simulink model "H175_Stage_01_Anode_Cathode"  (R2023a)
settings: Solver=VariableStepAuto  StartTime=0.0  StopTime=500  RelTol=1e-3
values from neighbouring files (symbols this model uses):
  anode_tube_D = 0.01    [All_Properties.mat]    (also in anode_subsystem_parameters.m; environment_parameters.m)
  D = 0.01    [All_Properties.mat]    (also in anode_subsystem_parameters.m)
  densityHydrogen = 0.0899    [All_Properties.mat]    (also in Valve_Init.m; anode_subsystem_parameters.m)
  Fischer_EMTC120K_supplier_mdot_TLU = [33.385172 57.11265182 82.35238332 173.9183787 230.2050798 50.1655574 86.1774137 122.96585 210.0188714 258.8737112 70.20710678 115.3896052 ... (25 elements, 5x5)]    [All_Properties.mat]    (also in cathode_subsystem_parameters.m = [33.385172 50.1655574 70.20710678 87.4902972 105.3161257)
  Fischer_EMTC120K_supplier_pr_TLU = [2.452176848 3.067593046 4.01020547 5.11549365 6.10066015 2.450765612 3.07166407 4.0616557 5.112468546 6.108742034 2.432340262 3.033516574 ... (25 elements, 5x5)]    [All_Properties.mat]    (also in cathode_subsystem_parameters.m = [2.452176848 2.450765612 2.432340262 2.407245766 2.37067916)
  Kv_VL6112 = 0.8    [All_Properties.mat]    (also in anode_subsystem_parameters.m)
  N2_T = [-56.55 -50 -40 -30 -20 -10 -5 -4 -3 -2 -1 0 ... (52 elements, 1x52)]    [All_Properties.mat]    (also in anode_subsystem_parameters.m = [-56.55 -50 -40 -30 -20 -10 -5 -4 -3 -2 -1 0 1 2 3 4 5 10 20; environment_parameters.m = [-56.55, -50:10:-10, -5:1:5, 10:10:350]; stack_model_harness_parameters.m = [-56.55, -50:10:-10, -5:1:5, 10:10:350])
  p_range = 0.005    [All_Properties.mat]    (also in anode_subsystem_parameters.m)
  r_max = 0.2    [All_Properties.mat]    (also in anode_subsystem_parameters.m)
  r_min = 0.0001    [All_Properties.mat]    (also in anode_subsystem_parameters.m)
  responseTimeValve = 0.013    [All_Properties.mat]    (also in anode_subsystem_parameters.m)
undefined symbols (not defined in the file or in its folder): sigbuilder_block
libraries: fl_lib x168, nesl_utility x116, SimscapeFluids_lib x8, slpidlib x5, simulink x1
(part 2 of 8)

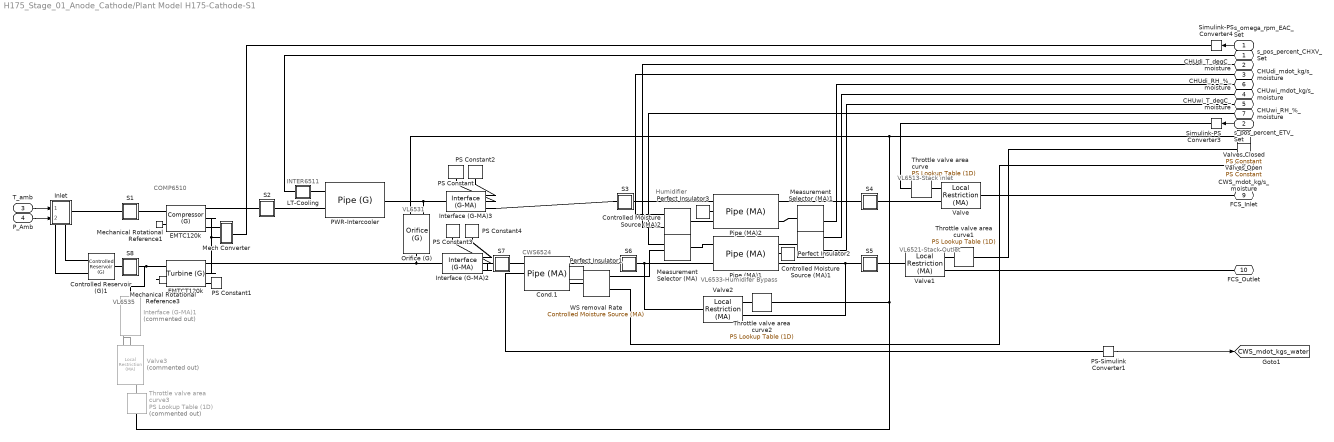
== system H175_Stage_01_Anode_Cathode/Plant Model H175-Cathode-S1 ==
  note: Humidifier
  note: COMP6510
  note: INTER6511
  note: VL6531
  note: VL6513-Stack inlet
  note: VL6521-Stack Outlet
  note: VL6533-Humidifer Bypass
  note: VL6535
  note: CWS6524
  s_omega_rpm_EAC_Set : Inport
  s_pos_percent_ETV_Set : Inport  Port=2
  T_amb : Inport  Port=3
  P_Amb : Inport  Port=4
  Cond.1 : fl_lib/Moist Air/Elements/Pipe (MA)  length=1 m  area=1 m^2  Dh=.1 m  length_add=.1 m  roughness=15e-6 m  Re_lam=2000  Re_tur=4000  shape_factor=64  Nu_lam=3.66  wall_condensation=simscape.enum.onoff.on  RH_ws=.2  time_constant=1e-3 s  moisture_trace_gas_source=foundation.enum.moisture_trace_gas_source.controlled  moisture_source_spec=foundation.enum.moisture_source_spec.vapor  moisture_mass_flow=0 kg/s  moisture_temperature_spec=foundation.enum.temperature_spec.atmospheric  moisture_temperature=293.15 K  trace_gas_mass_flow=0 kg/s  trace_gas_temperature_spec=foundation.enum.temperature_spec.atmospheric  trace_gas_temperature=293.15 K  p_I_specify=off  p_I_priority=High  p_I=0.101325 MPa  p_I_nominal_specify=off  p_I_nominal_unit=MPa  p_I_nominal_value=1  T_I_specify=off  T_I_priority=High  T_I=293.15 K  T_I_nominal_specify=off  T_I_nominal_unit=K  T_I_nominal_value=1  RH_I_specify=off  RH_I_priority=High  RH_I=0  RH_I_nominal_specify=off  RH_I_nominal_unit=1  RH_I_nominal_value=1  x_w_I_specify=off  x_w_I_priority=None  x_w_I=0  x_w_I_nominal_specify=off  x_w_I_nominal_unit=1  x_w_I_nominal_value=1  y_w_I_specify=off  y_w_I_priority=None  y_w_I=0  y_w_I_nominal_specify=off  y_w_I_nominal_unit=1  y_w_I_nominal_value=1  HR_I_specify=off  HR_I_priority=None  HR_I=0  HR_I_nominal_specify=off  HR_I_nominal_unit=1  HR_I_nominal_value=1  x_g_I_specify=off  x_g_I_priority=High  x_g_I=0  x_g_I_nominal_specify=off  x_g_I_nominal_unit=1  x_g_I_nominal_value=1  y_g_I_specify=off  y_g_I_priority=None  y_g_I=0  y_g_I_nominal_specify=off  y_g_I_nominal_unit=1  y_g_I_nominal_value=1
      settings: InternalSimscapePortConfiguration="{\"Bottom\":[],\"Left\":[{\"id\":\"A\",\"label\":\"A\",\"type\":\"foundation.moist_air.moist_air\"},{\"id\":\"H\",\"label\":\"H\",\"type\":\"foundation.thermal.thermal\"},{\"id\":\"S\",\"label\":\"S\",\"type\":\"foundation.moist_air.moist_air_source\"}],\"Right\":[{\"id\":\"B\",\"label\":\"B\",\"type\":\"foundation.moist_air.moist_air\"},{\"id\":\"W\",\"label\":\"W\",\"type\":\"output\"},{\"id\":\"F\",\"label\":\"F\",\"type\":\"output\"}],\"Top\":[]}"
  Controlled Moisture Source (MA)1 : fl_lib/Moist Air/Sources/Moisture & Trace Gas Sources/Controlled Moisture Source (MA)  moisture_source_spec=foundation.enum.moisture_source_spec.vapor  Phi_S_specify=off  Phi_S_priority=None  Phi_S=0 kW  Phi_S_nominal_specify=off  Phi_S_nominal_unit=kW  Phi_S_nominal_value=1  mdot_w_S_specify=off  mdot_w_S_priority=None  mdot_w_S=0 kg/s  mdot_w_S_nominal_specify=off  mdot_w_S_nominal_unit=kg/s  mdot_w_S_nominal_value=1
      settings: InternalSimscapePortConfiguration="{\"Bottom\":[],\"Left\":[{\"id\":\"S\",\"label\":\"S\",\"type\":\"foundation.moist_air.moist_air_source\"}],\"Right\":[{\"id\":\"M\",\"label\":\"M\",\"type\":\"input\"},{\"id\":\"T\",\"label\":\"T\",\"type\":\"input\"}],\"Top\":[]}"
  Controlled Moisture Source (MA)2 : fl_lib/Moist Air/Sources/Moisture & Trace Gas Sources/Controlled Moisture Source (MA)  moisture_source_spec=foundation.enum.moisture_source_spec.vapor  Phi_S_specify=off  Phi_S_priority=None  Phi_S=0 kW  Phi_S_nominal_specify=off  Phi_S_nominal_unit=kW  Phi_S_nominal_value=1  mdot_w_S_specify=off  mdot_w_S_priority=None  mdot_w_S=0 kg/s  mdot_w_S_nominal_specify=off  mdot_w_S_nominal_unit=kg/s  mdot_w_S_nominal_value=1
      settings: InternalSimscapePortConfiguration="{\"Bottom\":[],\"Left\":[{\"id\":\"S\",\"label\":\"S\",\"type\":\"foundation.moist_air.moist_air_source\"}],\"Right\":[{\"id\":\"M\",\"label\":\"M\",\"type\":\"input\"},{\"id\":\"T\",\"label\":\"T\",\"type\":\"input\"}],\"Top\":[]}"
  Controlled Reservoir (G)1 : fl_lib/Gas/Elements/Controlled Reservoir (G)  area_A=0.002 m^2
      settings: InternalSimscapePortConfiguration="{\"Bottom\":[],\"Left\":[{\"id\":\"A\",\"label\":\"A\",\"type\":\"foundation.gas.gas\"}],\"Right\":[{\"id\":\"T_in\",\"label\":\"T\",\"type\":\"input\"},{\"id\":\"p_in\",\"label\":\"P\",\"type\":\"input\"}],\"Top\":[]}"
  EMTC120k : SimscapeFluids_lib/Gas/Turbomachinery/Compressor (G)  parameterization=fluids.gas.turbomachinery.enum.CompressorParameterization.Tabulated  NDes=10000 rpm  piDes=7.5  mdotDes=33 kg/s  efficiencyType=fluids.gas.turbomachinery.enum.EfficiencyType.Analytical  efficiencyValue=0.8  etaMax=0.887  etaMin=0.5  mdotMaxEff=30 kg/s  piMaxEff=7  omega_TLU=Fischer_EMTC120K_supplier_omega_TLU rpm  beta_TLU=Fischer_EMTC120K_supplier_beta_TLU  pr_TLU=Fischer_EMTC120K_supplier_pr_TLU/2  mdot_TLU=Fischer_EMTC120K_supplier_mdot_TLU/2 g/s  eta_TLU=Fischer_EMTC120K_supplier_eta_TLU  SMFault=simscape.enum.assert.action.none  a=1.5  b=5  k=0.03  c=3  d=4  cCap=15  dCap=1.0  p_reference=0.101325 MPa  T_reference=288.15 K  mechanical_efficiency=0.98  area_A=.002 m^2  area_B=.002 m^2
      settings: LogSimulationData=on  InternalSimscapePortConfiguration="{\"Bottom\":[],\"Left\":[{\"id\":\"A\",\"label\":\"A\",\"type\":\"foundation.gas.gas\"},{\"id\":\"C\",\"label\":\"C\",\"type\":\"foundation.mechanical.rotational.rotational\"}],\"Right\":[{\"id\":\"B\",\"label\":\"B\",\"type\":\"foundation.gas.gas\"},{\"id\":\"R\",\"label\":\"R\",\"type\":\"foundation.mechanical.rotational.rotational\"},{\"id\":\"SM\",\"label\":\"SM\",\"type\":\"output\"}],\"Top\":[]}"
  EMTCT120k : SimscapeFluids_lib/Gas/Turbomachinery/Turbine (G)  parameterization=fluids.gas.turbomachinery.enum.TurbineParameterization.Tabulated1D  omega_TLU_2=[31000, 45000, 60000, 75000, 90000, 105000, 120000] rpm  variable_nozzle=true  min_nozzle_opening=1e-3  max_nozzle_opening=1  pr_nom=2  mdot_nom=0.08 kg/s  pr_mdot_TLU=[1.1667,1.405,1.791,2.18,2.5194]  mdot_TLU=[.0527,.08728,.1276,.1668,.1927] kg/s  pr_mdot_TLU_2=[1.217, 1.285, 1.323, 1.363, 1.402, 1.427, 1.495, 1.545, 1.6, 1.687, 1.747, 1.8074; 1.231, 1.302, 1.356, 1.404, 1.443, 1.473, 1.525, 1.577, 1.635, 1.709, 1.782, 1.845; 1.242, 1.328, 1.388, 1.437, 1.528, 1.617, 1.704, 1.811, 1.915, 1.979, 2.053, 2.1226; 1.244, 1.339, 1.417, 1.465, 1.528, 1.584, 1.692, 1.787, 1.899, 2, 2.075, 2.1492; 1.245, 1.34, 1.425, 1.492, 1.546, 1.684, 1.748, 1.882, 1.987, 2.084, 2.167, 2.2458; 1.251, 1.345, 1.442, 1.521, 1.596, 1.692, 1.849, 1.972, 2.1, 2.173, 2.259, 2.3424; 1.248, 1.348, 1.447, 1.516, 1.581, 1.651, 1.749, 1.839, 1.93, 2.024, 2.154, 2.242]  mdot_TLU_2=[40.403, 44.417, 46.653, 47.966, 48.97, 49.544, 50.001, 50.081, 50.086, 50.095, 50.09, 50.0922; 40.044, 43.754, 46.125, 47.626, 48.513, 49.105, 49.481, 49.58, 49.597, 49.624, 49.638, 49.633; 39.941, 43.795, 46.017, 47.335, 48.795, 49.199, 49.279, 49.27, 49.248, 49.23, 49.255, 49.2428; 39.896, 43.512, 45.914, 47.061, 48.011, 48.558, 48.943, 49.042, 49.069, 49.01, 49.046, 49.0266; 39.524, 42.934, 45.686, 46.743, 47.715, 48.67, 48.777, 48.836, 48.876, 48.836, 48.845, 48.8184; 39.439, 43.01, 45.556, 46.801, 47.792, 48.388, 48.634, 48.67, 48.639, 48.647, 48.625, 48.5912; 39.502, 42.849, 45.336, 46.385, 47.312, 47.877, 48.222, 48.397, 48.459, 48.482, 48.455, 48.414] kg/s  efficiency_constant=.954  pr_eta_TLU=[1.1667,1.405,1.791,2.18,2.5194]  eta_TLU=[0.6804,.76609,.7634,.7426,.72]  pr_eta_TLU_2=[1.224, 1.246, 1.292, 1.387, 1.457, 1.534, 1.61, 1.686, 1.743, 1.79, 1.871, 1.914; 1.237, 1.25, 1.28, 1.369, 1.459, 1.553, 1.629, 1.716, 1.799, 1.846, 1.927, 1.97; 1.241, 1.255, 1.283, 1.326, 1.401, 1.509, 1.591, 1.704, 1.806, 1.913, 1.994, 2.037; 1.25, 1.265, 1.308, 1.364, 1.456, 1.532, 1.637, 1.739, 1.851, 1.934, 2.042, 2.085; 1.281, 1.314, 1.371, 1.425, 1.498, 1.574, 1.647, 1.749, 1.878, 1.979, 2.091, 2.18; 1.252, 1.328, 1.425, 1.544, 1.642, 1.757, 1.873, 2.005, 2.1, 2.204, 2.248, 2.28; 1.382, 1.43, 1.495, 1.586, 1.688, 1.791, 1.887, 1.99, 2.079, 2.158, 2.249, 2.36]  eta_TLU_2=[.72, .754, .759, .739, .714, .679, .643, .603, .554, .524, .494, .48; .716, .757, .794, .819, .812, .788, .761, .728, .692, .662, .632, .618; .629, .691, .775, .831, .858, .869, .859, .842, .816, .782, .752, .738; .594, .668, .757, .804, .857, .883, .892, .893, .884, .865, .835, .821; .664, .72, .779, .823, .858, .883, .897, .905, .904, .896, .883, .868; .559, .61, .673, .741, .788, .835, .869, .895, .908, .899, .854, .751; .718, .785, .824, .855, .882, .9, .908, .906, .884, .857, .804, .701]  p_reference=1.8 bar  T_reference=85 degC  mechanical_efficiency=0.98  area_A=0.002 m^2  area_B=0.002 m^2
      settings: LogSimulationData=on  InternalSimscapePortConfiguration="{\"Bottom\":[],\"Left\":[{\"id\":\"A\",\"label\":\"A\",\"type\":\"foundation.gas.gas\"},{\"id\":\"R\",\"label\":\"R\",\"type\":\"foundation.mechanical.rotational.rotational\"},{\"id\":\"VN\",\"label\":\"VN\",\"type\":\"input\"}],\"Right\":[{\"id\":\"B\",\"label\":\"B\",\"type\":\"foundation.gas.gas\"},{\"id\":\"C\",\"label\":\"C\",\"type\":\"foundation.mechanical.rotational.rotational\"}],\"Top\":[]}"
  Inlet : Subsystem
      settings: PortSchema="{\"entries\":[{\"content\":{\"sides\":[{\"content\":{\"connectorIds\":[\"In1\",\"In2\"]},\"type\":\"ConnectorPlacement.EquallySpacedRectSide\",\"uuid\":\"383c8b90-d22b-483c-be09-d78d9bde0881\"},{\"content\":{\"connectorIds\":[\"RConn1\"],\"side\":\"RIGHT\"},\"type\":\"ConnectorPlacement.EquallySpacedRectSide\",\"uuid\":\"3dc3e004-4331-4c40-8051-329aa9250422\"},{\"content\":{\"side\":\"TOP\"},\"type\":\"ConnectorPlacement.EquallySpacedRectSide\",\"uuid\":\"aff35d8f-ac03-451a-b72e-dc7bd89924e8\"},{\"content\":{\"connectorIds\":[\"RConn2\",\"RConn3\"],\"side\":\"BOTTOM\"},\"type\":\"ConnectorPlacement.EquallySpacedRectSide\",\"uuid\":\"82493911-a5c4-468a-a003-983b92ffd105\"}]},\"type\":\"ConnectorPlacement.EquallySpacedConnector\",\"uuid\":\"d9a1e9aa-22f5-4e42-bf15-8a8ecd9f58f9\"}],\"packageUris\":[\"http://schema.mathworks.com/mf0/Connector/R2020b\"],\"version\":\"1.0\"}"
  Interface (G-MA)1 : SimscapeFluids_lib/Fluid Network Interfaces/Interface (G-MA)  Commented=on  interface_type=foundation.enum.constant_controlled.controlled  moisture_spec=foundation.enum.moisture_spec.relative_humidity  RH_interface=0.5  x_w_interface=0.01  y_w_interface=0.01  HR_interface=0.01  Tw_interface=287 K  trace_gas_spec=foundation.enum.trace_gas_spec.mass_fraction  x_g_interface=1  y_g_interface=0.001  RH_ws=1  area=0.01 m^2  input_error_spec=foundation.enum.input_range_error.warn
      settings: InternalSimscapePortConfiguration="{\"Bottom\":[{\"id\":\"W\",\"label\":\"W\",\"type\":\"input\"},{\"id\":\"TG\",\"label\":\"TG\",\"type\":\"input\"}],\"Left\":[{\"id\":\"G\",\"label\":\"G\",\"type\":\"foundation.gas.gas\"}],\"Right\":[{\"id\":\"MA\",\"label\":\"MA\",\"type\":\"foundation.moist_air.moist_air\"}],\"Top\":[]}"
  Interface (G-MA)2 : SimscapeFluids_lib/Fluid Network Interfaces/Interface (G-MA)  interface_type=foundation.enum.constant_controlled.controlled  moisture_spec=foundation.enum.moisture_spec.relative_humidity  RH_interface=0.5  x_w_interface=0.01  y_w_interface=0.01  HR_interface=0.01  Tw_interface=287 K  trace_gas_spec=foundation.enum.trace_gas_spec.mass_fraction  x_g_interface=1  y_g_interface=0.001  RH_ws=1  area=0.01 m^2  input_error_spec=foundation.enum.input_range_error.warn
      settings: InternalSimscapePortConfiguration="{\"Bottom\":[{\"id\":\"W\",\"label\":\"W\",\"type\":\"input\"},{\"id\":\"TG\",\"label\":\"TG\",\"type\":\"input\"}],\"Left\":[{\"id\":\"G\",\"label\":\"G\",\"type\":\"foundation.gas.gas\"}],\"Right\":[{\"id\":\"MA\",\"label\":\"MA\",\"type\":\"foundation.moist_air.moist_air\"}],\"Top\":[]}"
  Interface (G-MA)3 : SimscapeFluids_lib/Fluid Network Interfaces/Interface (G-MA)  interface_type=foundation.enum.constant_controlled.controlled  moisture_spec=foundation.enum.moisture_spec.relative_humidity  RH_interface=0.5  x_w_interface=0.01  y_w_interface=0.01  HR_interface=0.01  Tw_interface=287 K  trace_gas_spec=foundation.enum.trace_gas_spec.mass_fraction  x_g_interface=1  y_g_interface=0.001  RH_ws=1  area=0.002 m^2  input_error_spec=foundation.enum.input_range_error.warn
      settings: InternalSimscapePortConfiguration="{\"Bottom\":[{\"id\":\"W\",\"label\":\"W\",\"type\":\"input\"},{\"id\":\"TG\",\"label\":\"TG\",\"type\":\"input\"}],\"Left\":[{\"id\":\"G\",\"label\":\"G\",\"type\":\"foundation.gas.gas\"}],\"Right\":[{\"id\":\"MA\",\"label\":\"MA\",\"type\":\"foundation.moist_air.moist_air\"}],\"Top\":[]}"
  LT-Cooling : Subsystem
  Measurement Selector (MA) : fl_lib/Moist Air/Sensors/Measurement Selector (MA)  moisture_spec=foundation.enum.moisture_spec.relative_humidity  trace_gas_spec=foundation.enum.trace_gas_spec.mole_fraction
  Measurement Selector (MA)1 : fl_lib/Moist Air/Sensors/Measurement Selector (MA)  moisture_spec=foundation.enum.moisture_spec.relative_humidity  trace_gas_spec=foundation.enum.trace_gas_spec.mole_fraction
  Mech Converter : Subsystem
  Mechanical Rotational Reference1 : fl_lib/Mechanical/Rotational Elements/Mechanical Rotational Reference
  Mechanical Rotational Reference3 : fl_lib/Mechanical/Rotational Elements/Mechanical Rotational Reference
  Orifice (G) : SimscapeFluids_lib/Gas/Valves & Orifices/Orifice (G)  orifice_type=foundation.enum.constant_variable.variable  orifice_parameterization=fluids.gas.valves_orifices.enum.OrificeParameterization.Area  opening_characteristic=fluids.gas.valves_orifices.enum.OpeningCharacteristics.Tabulated  Cv_constant=4  Cv_max=.369  L_Cv_TLU=0 : 0.2 : 1  Cv_TLU=[1e-06, .8, 1.6, 2.4, 3.2, 4]  xT_Cv=0.35  Kv_constant=3.6  Kv_max=50  L_Kv_TLU=[0,.15, .25, .35, .5, 1]  Kv_TLU=[1,27.76,115.14,223.57,336.62,462.54]  xT_Kv=.027  C_constant=12 l/(bar*s)  B_crit_constant=0.3  C_max=40 l/(bar*s)  B_crit_linear=0.25  L_C_TLU=0 : 0.2 : 1  C_TLU=[1e-05, 2.4, 4.8, 7.2, 9.6, 12] l/(bar*s)  B_crit_TLU=0.3 * ones(1, 6)  m=0.5  T_ref_C=293.15 K  rho_ref_C=1.185 kg/m^3  orifice_area_constant=1e-4 m^2  orifice_area_max=0.00152 m^2  L_orifice_area_TLU=[0.111111111,0.222222222,0.333333333,0.444444444,0.555555556,0.666666667,0.777777778,0.888888889,1]  orifice_area_TLU=[2.00E-08,9.00E-08,0.0002,0.00035,0.00055,0.00077,0.00101,0.00125,0.00153] m^2  Cd=.64  leakage_fraction=0.03185  smoothing_factor=0.01  B_lam=9.44E-01  area=0.002 m^2
      settings: InternalSimscapePortConfiguration="{\"Bottom\":[],\"Left\":[{\"id\":\"A\",\"label\":\"A\",\"type\":\"foundation.gas.gas\"},{\"id\":\"L\",\"label\":\"L\",\"type\":\"input\"}],\"Right\":[{\"id\":\"B\",\"label\":\"B\",\"type\":\"foundation.gas.gas\"}],\"Top\":[]}"
  PS Constant : fl_lib/Physical Signals/Sources/PS Constant  constant=.2
  PS Constant1 : fl_lib/Physical Signals/Sources/PS Constant  constant=1
  PS Constant2 : fl_lib/Physical Signals/Sources/PS Constant  constant=.001
  PS Constant3 : fl_lib/Physical Signals/Sources/PS Constant  constant=.3
  PS Constant4 : fl_lib/Physical Signals/Sources/PS Constant  constant=.001
  PS-Simulink Converter1 : nesl_utility/PS-Simulink Converter  PhysicalDomain=network_engine_domain  SubClassName=ps_output  LeftPortType=input  RightPortType=output  PseudoPeriodic=off  Frequencies=[]  VectorFormat=inherit  Unit=inherit  AffineConversion=off
  PWR-Intercooler : fl_lib/Gas/Elements/Pipe (G)  length=1 m  area=1 m^2  Dh=0.1 m  length_add=.2 m  roughness=15e-14 m  Re_lam=2000  Re_tur=4000  shape_factor=3.66  Nu_lam=150  p_I_specify=off  p_I_priority=High  p_I=1.8 bar  p_I_nominal_specify=off  p_I_nominal_unit=MPa  p_I_nominal_value=.1  T_I_specify=off  T_I_priority=High  T_I=293.15 K  T_I_nominal_specify=off  T_I_nominal_unit=K  T_I_nominal_value=1  rho_I_specify=off  rho_I_priority=None  rho_I=1.2 kg/m^3  rho_I_nominal_specify=off  rho_I_nominal_unit=kg/m^3  rho_I_nominal_value=1
      settings: LogSimulationData=on
  Perfect Insulator1 : fl_lib/Thermal/Thermal Elements/Perfect Insulator  T_specify=off  T_priority=None  T=293.15 K  T_nominal_specify=off  T_nominal_unit=K  T_nominal_value=1
  Perfect Insulator2 : fl_lib/Thermal/Thermal Elements/Perfect Insulator  T_specify=off  T_priority=None  T=0 K  T_nominal_specify=off  T_nominal_unit=K  T_nominal_value=1
  Perfect Insulator3 : fl_lib/Thermal/Thermal Elements/Perfect Insulator  T_specify=off  T_priority=None  T=0 K  T_nominal_specify=off  T_nominal_unit=K  T_nominal_value=1
  Pipe (MA)1 : fl_lib/Moist Air/Elements/Pipe (MA)  length=0.25 m  area=pi*0.05^2/4 m^2  Dh=0.05 m  length_add=0.1 m  roughness=15e-6 m  Re_lam=2000  Re_tur=4000  shape_factor=64  Nu_lam=3.66  wall_condensation=simscape.enum.onoff.off  RH_ws=1  time_constant=1e-3 s  moisture_trace_gas_source=foundation.enum.moisture_trace_gas_source.controlled  moisture_source_spec=foundation.enum.moisture_source_spec.vapor  moisture_mass_flow=0 kg/s  moisture_temperature_spec=foundation.enum.temperature_spec.atmospheric  moisture_temperature=293.15 K  trace_gas_mass_flow=0 kg/s  trace_gas_temperature_spec=foundation.enum.temperature_spec.atmospheric  trace_gas_temperature=293.15 K  p_I_specify=off  p_I_priority=High  p_I=env_p MPa  p_I_nominal_specify=off  p_I_nominal_unit=MPa  p_I_nominal_value=1  T_I_specify=off  T_I_priority=High  T_I=env_T degC  T_I_nominal_specify=off  T_I_nominal_unit=K  T_I_nominal_value=1  RH_I_specify=off  RH_I_priority=High  RH_I=env_RH  RH_I_nominal_specify=off  RH_I_nominal_unit=1  RH_I_nominal_value=1  x_w_I_specify=off  x_w_I_priority=None  x_w_I=0  x_w_I_nominal_specify=off  x_w_I_nominal_unit=1  x_w_I_nominal_value=1  y_w_I_specify=off  y_w_I_priority=None  y_w_I=0  y_w_I_nominal_specify=off  y_w_I_nominal_unit=1  y_w_I_nominal_value=1  HR_I_specify=off  HR_I_priority=None  HR_I=0  HR_I_nominal_specify=off  HR_I_nominal_unit=1  HR_I_nominal_value=1  x_g_I_specify=off  x_g_I_priority=None  x_g_I=0  x_g_I_nominal_specify=off  x_g_I_nominal_unit=1  x_g_I_nominal_value=1  y_g_I_specify=off  y_g_I_priority=High  y_g_I=env_yO2  y_g_I_nominal_specify=off  y_g_I_nominal_unit=1  y_g_I_nominal_value=1
      settings: InternalSimscapePortConfiguration="{\"Bottom\":[],\"Left\":[{\"id\":\"A\",\"label\":\"A\",\"type\":\"foundation.moist_air.moist_air\"},{\"id\":\"H\",\"label\":\"H\",\"type\":\"foundation.thermal.thermal\"},{\"id\":\"S\",\"label\":\"S\",\"type\":\"foundation.moist_air.moist_air_source\"}],\"Right\":[{\"id\":\"B\",\"label\":\"B\",\"type\":\"foundation.moist_air.moist_air\"},{\"id\":\"W\",\"label\":\"W\",\"type\":\"output\"},{\"id\":\"F\",\"label\":\"F\",\"type\":\"output\"}],\"Top\":[]}"
  Pipe (MA)2 : fl_lib/Moist Air/Elements/Pipe (MA)  length=0.25 m  area=pi*0.05^2/4 m^2  Dh=0.05 m  length_add=0.1 m  roughness=15e-6 m  Re_lam=2000  Re_tur=4000  shape_factor=64  Nu_lam=3.66  wall_condensation=simscape.enum.onoff.off  RH_ws=1  time_constant=1e-3 s  moisture_trace_gas_source=foundation.enum.moisture_trace_gas_source.controlled  moisture_source_spec=foundation.enum.moisture_source_spec.vapor  moisture_mass_flow=0 kg/s  moisture_temperature_spec=foundation.enum.temperature_spec.atmospheric  moisture_temperature=293.15 K  trace_gas_mass_flow=0 kg/s  trace_gas_temperature_spec=foundation.enum.temperature_spec.atmospheric  trace_gas_temperature=293.15 K  p_I_specify=off  p_I_priority=High  p_I=env_p MPa  p_I_nominal_specify=off  p_I_nominal_unit=MPa  p_I_nominal_value=1  T_I_specify=on  T_I_priority=High  T_I=env_T degC  T_I_nominal_specify=off  T_I_nominal_unit=K  T_I_nominal_value=1  RH_I_specify=on  RH_I_priority=High  RH_I=env_RH  RH_I_nominal_specify=off  RH_I_nominal_unit=1  RH_I_nominal_value=1  x_w_I_specify=off  x_w_I_priority=None  x_w_I=0  x_w_I_nominal_specify=off  x_w_I_nominal_unit=1  x_w_I_nominal_value=1  y_w_I_specify=off  y_w_I_priority=None  y_w_I=0  y_w_I_nominal_specify=off  y_w_I_nominal_unit=1  y_w_I_nominal_value=1  HR_I_specify=off  HR_I_priority=None  HR_I=0  HR_I_nominal_specify=off  HR_I_nominal_unit=1  HR_I_nominal_value=1  x_g_I_specify=off  x_g_I_priority=None  x_g_I=0  x_g_I_nominal_specify=off  x_g_I_nominal_unit=1  x_g_I_nominal_value=1  y_g_I_specify=off  y_g_I_priority=High  y_g_I=env_yO2  y_g_I_nominal_specify=off  y_g_I_nominal_unit=1  y_g_I_nominal_value=1
      settings: InternalSimscapePortConfiguration="{\"Bottom\":[],\"Left\":[{\"id\":\"A\",\"label\":\"A\",\"type\":\"foundation.moist_air.moist_air\"},{\"id\":\"H\",\"label\":\"H\",\"type\":\"foundation.thermal.thermal\"},{\"id\":\"S\",\"label\":\"S\",\"type\":\"foundation.moist_air.moist_air_source\"}],\"Right\":[{\"id\":\"B\",\"label\":\"B\",\"type\":\"foundation.moist_air.moist_air\"},{\"id\":\"W\",\"label\":\"W\",\"type\":\"output\"},{\"id\":\"F\",\"label\":\"F\",\"type\":\"output\"}],\"Top\":[]}"
  S1 : Subsystem
  S2 : Subsystem
  S3 : Subsystem
  S4 : Subsystem
  S5 : Subsystem
  S6 : Subsystem
  S7 : Subsystem
  S8 : Subsystem
  Simulink-PS Converter3 : nesl_utility/Simulink-PS Converter  PhysicalDomain=network_engine_domain  SubClassName=ps_input  LeftPortType=input  RightPortType=output  PseudoPeriodic=off  Frequencies=[]  NoiseDistribution=none  NoiseParameters=[]  Unit=1  AffineConversion=off  FilteringAndDerivatives=provide  SimscapeFilterOrder=1  InputFilterTimeConstant=0.001  UdotUserProvided=0
  Simulink-PS Converter4 : nesl_utility/Simulink-PS Converter  PhysicalDomain=network_engine_domain  SubClassName=ps_input  LeftPortType=input  RightPortType=output  PseudoPeriodic=off  Frequencies=[]  NoiseDistribution=none  NoiseParameters=[]  Unit=1  AffineConversion=off  FilteringAndDerivatives=provide  SimscapeFilterOrder=1  InputFilterTimeConstant=0.001  UdotUserProvided=0
  Throttle valve area curve : fl_lib/Physical Signals/Lookup Tables/PS Lookup Table (1D)  x=[0,.2,.3,.4,.5,.6,.7,.8,.9,1]  f=[0.000011,0.00002,0.00009,0.00020,0.00035,0.00055,0.00077,0.00101,0.00125,0.00153]  interp_method=simscape.enum.interpolation.smooth  extrap_method=simscape.enum.extrapolation.linear
  Throttle valve area curve1 : fl_lib/Physical Signals/Lookup Tables/PS Lookup Table (1D)  x=[0,.2,.3,.4,.5,.6,.7,.8,.9,1]  f=[0.000011,0.00002,0.00009,0.00020,0.00035,0.00055,0.00077,0.00101,0.00125,0.00153]  interp_method=simscape.enum.interpolation.smooth  extrap_method=simscape.enum.extrapolation.linear
  Throttle valve area curve2 : fl_lib/Physical Signals/Lookup Tables/PS Lookup Table (1D)  x=[0,.2,.3,.4,.5,.6,.7,.8,.9,1]  f=[0.0000011,0.000002,0.00009,0.00020,0.00035,0.00055,0.00077,0.00101,0.00125,0.00153]  interp_method=simscape.enum.interpolation.smooth  extrap_method=simscape.enum.extrapolation.linear
  Throttle valve area curve3 : fl_lib/Physical Signals/Lookup Tables/PS Lookup Table (1D)  Commented=on  x=[0,.2,.3,.4,.5,.6,.7,.8,.9,1]  f=[0.000011,0.00002,0.00009,0.00020,0.00035,0.00055,0.00077,0.00101,0.00125,0.00153]  interp_method=simscape.enum.interpolation.smooth  extrap_method=simscape.enum.extrapolation.linear
  Valve : fl_lib/Moist Air/Elements/Local Restriction (MA)  restriction_type=foundation.enum.restriction_type.variable  restriction_area=0.001 m^2  min_area=2e-5 m^2  max_area=.00165 m^2  area=.002 m^2  Cd=3.5  B_lam=9.44E-01
  Valve1 : fl_lib/Moist Air/Elements/Local Restriction (MA)  restriction_type=foundation.enum.restriction_type.variable  restriction_area=0.001 m^2  min_area=2e-5 m^2  max_area=.00165 m^2  area=.002 m^2  Cd=3.5  B_lam=9.44E-01
  Valve2 : fl_lib/Moist Air/Elements/Local Restriction (MA)  restriction_type=foundation.enum.restriction_type.variable  restriction_area=0.001 m^2  min_area=2e-5 m^2  max_area=.00165 m^2  area=.002 m^2  Cd=3.5  B_lam=9.44E-01
  Valve3 : fl_lib/Moist Air/Elements/Local Restriction (MA)  Commented=on  restriction_type=foundation.enum.restriction_type.variable  restriction_area=0.001 m^2  min_area=2e-5 m^2  max_area=.00153 m^2  area=.002 m^2  Cd=3.5  B_lam=9.44E-01
  Valves Closed : fl_lib/Physical Signals/Sources/PS Constant  constant=0
  Valves Open : fl_lib/Physical Signals/Sources/PS Constant  constant=1
  WS removal Rate : fl_lib/Moist Air/Sources/Moisture & Trace Gas Sources/Controlled Moisture Source (MA)  moisture_source_spec=foundation.enum.moisture_source_spec.liquid  Phi_S_specify=off  Phi_S_priority=None  Phi_S=0 kW  Phi_S_nominal_specify=off  Phi_S_nominal_unit=kW  Phi_S_nominal_value=1  mdot_w_S_specify=off  mdot_w_S_priority=None  mdot_w_S=0 kg/s  mdot_w_S_nominal_specify=off  mdot_w_S_nominal_unit=kg/s  mdot_w_S_nominal_value=1
      settings: InternalSimscapePortConfiguration="{\"Bottom\":[],\"Left\":[{\"id\":\"S\",\"label\":\"S\",\"type\":\"foundation.moist_air.moist_air_source\"}],\"Right\":[{\"id\":\"M\",\"label\":\"M\",\"type\":\"input\"},{\"id\":\"T\",\"label\":\"T\",\"type\":\"input\"}],\"Top\":[]}"
  s_pos_percent_CHXV_Set : PMIOPort  Side=Left
  CHUdi_T_degC_moisture : PMIOPort  Port=2  Side=Left
  CHUdi_mdot_kg/s_moisture : PMIOPort  Port=3  Side=Left
  CHUwi_mdot_kg/s_moisture : PMIOPort  Port=4  Side=Left
  CHUwi_T_degC_moisture : PMIOPort  Port=5  Side=Left
  CHUdi_RH_%_moisture : PMIOPort  Port=6  Side=Left
  CHUwi_RH_%_moisture : PMIOPort  Port=7  Side=Left
  CWS_mdot_kg/s_moisture : PMIOPort  Port=8  Side=Left
  FCS_Inlet : PMIOPort  Port=9  Side=Right
  FCS_Outlet : PMIOPort  Port=10  Side=Right
  tag scope: CWS_mdot_kgs_water=global
  wires:
  P_Amb/1 -> Inlet/2(Inport1)
  T_amb/1 -> Inlet/1(Inport)
  s_omega_rpm_EAC_Set/1 -> Simulink-PS Converter4/1
  s_pos_percent_ETV_Set/1 -> Simulink-PS Converter3/1
  PS-Simulink Converter1/1 -> [CWS_mdot_kgs_water]
  connections:
  EMTCT120k/LConn3 -- PS Constant1/RConn1
  Controlled Reservoir (G)1/RConn2 -- Inlet/RConn2
  S2/RConn1 -- PWR-Intercooler/LConn1
  S1/LConn1 -- Inlet/RConn1
  EMTCT120k/RConn2 -- Mechanical Rotational Reference3/LConn1
  Controlled Reservoir (G)1/RConn1 -- Inlet/RConn3
  EMTC120k/RConn1 -- S2/LConn1
  EMTC120k/RConn3 -- Mech Converter/LConn1
  EMTC120k/LConn1 -- S1/RConn1
  Interface (G-MA)3/RConn3 -- PS Constant2/RConn1
  Interface (G-MA)2/RConn3 -- PS Constant4/RConn1
  Interface (G-MA)3/RConn2 -- PS Constant/RConn1
  Interface (G-MA)2/RConn2 -- PS Constant3/RConn1
  EMTC120k/LConn2 -- Mechanical Rotational Reference1/LConn1
  Interface (G-MA)3/RConn1 -- S3/RConn1
  Orifice (G)/LConn1 -- PWR-Intercooler/RConn1 -- Interface (G-MA)3/LConn1
  Valves Open/RConn1 -- Throttle valve area curve1/LConn1
  FCS_Inlet/RConn1 -- Valve/RConn1
  EMTC120k/RConn2 -- EMTCT120k/LConn2 -- Mech Converter/LConn2
  Mech Converter/RConn1 -- Simulink-PS Converter4/RConn1
  s_pos_percent_CHXV_Set/RConn1 -- LT-Cooling/LConn1
  PWR-Intercooler/LConn2 -- LT-Cooling/RConn1
  EMTCT120k/RConn1 -- Interface (G-MA)1/LConn1 -- S8/LConn1
  Controlled Reservoir (G)1/LConn1 -- S8/RConn1
  Orifice (G)/RConn1 -- EMTCT120k/LConn1 -- Interface (G-MA)2/LConn1
  Valve/LConn2 -- Throttle valve area curve/RConn1
  Simulink-PS Converter3/RConn1 -- Throttle valve area curve/LConn1
  S4/LConn1 -- Valve/LConn1
  Valve1/LConn2 -- Throttle valve area curve1/RConn1
  Valve1/RConn1 -- S5/LConn1
  Valves Closed/RConn1 -- Throttle valve area curve2/LConn1 -- Throttle valve area curve3/LConn1 -- Orifice (G)/LConn2
  Valve2/LConn2 -- Throttle valve area curve2/RConn1
  Valve3/LConn2 -- Throttle valve area curve3/RConn1
  Interface (G-MA)1/RConn1 -- Valve3/RConn1
  WS removal Rate/LConn1 -- Cond.1/LConn3
  Pipe (MA)2/LConn1 -- S3/LConn1
  Controlled Moisture Source (MA)1/LConn1 -- Pipe (MA)1/LConn3
  Measurement Selector (MA)/RConn3 -- CHUwi_RH_%_moisture/RConn1
  Perfect Insulator2/LConn1 -- Pipe (MA)1/LConn2
  Measurement Selector (MA)/LConn1 -- Pipe (MA)1/RConn3
  Controlled Moisture Source (MA)1/RConn2 -- CHUwi_mdot_kg/s_moisture/RConn1
  Measurement Selector (MA)1/LConn1 -- Pipe (MA)2/RConn3
  Perfect Insulator3/LConn1 -- Pipe (MA)2/LConn2
  Controlled Moisture Source (MA)2/LConn1 -- Pipe (MA)2/LConn3
  CHUdi_mdot_kg/s_moisture/RConn1 -- Controlled Moisture Source (MA)2/RConn1
  Controlled Moisture Source (MA)2/RConn2 -- CHUdi_T_degC_moisture/RConn1
  Measurement Selector (MA)1/RConn3 -- CHUdi_RH_%_moisture/RConn1
  CHUwi_T_degC_moisture/RConn1 -- Controlled Moisture Source (MA)1/RConn1
  Pipe (MA)1/RConn1 -- Valve2/RConn1 -- S6/LConn1
  Pipe (MA)1/LConn1 -- S5/RConn1 -- Valve2/LConn1
  Interface (G-MA)2/RConn1 -- S7/RConn1
  S7/LConn1 -- Cond.1/RConn1
  CWS_mdot_kg/s_moisture/RConn1 -- WS removal Rate/RConn1
  Perfect Insulator1/LConn1 -- Cond.1/LConn2
  Pipe (MA)2/RConn1 -- S4/RConn1
  FCS_Outlet/RConn1 -- Valve1/LConn1
  S6/RConn1 -- Cond.1/LConn1
  WS removal Rate/RConn2 -- Measurement Selector (MA)/RConn2
  Cond.1/RConn2 -- PS-Simulink Converter1/LConn1

== system H175_Stage_01_Anode_Cathode/Power2Current ==
  In1 : Inport
  Power2I : Lookup_n-D  NumberOfTableDimensions=1  BreakpointsForDimension1=[0;8.5;17;26;34;42;50;58.3;66.66;85;100]  Table=[0;50;100;150;200;250;300;350;400;510;600]  InternalRulePriority=Speed  RndMeth=Simplest
  Power2I1 : Lookup_n-D  NumberOfTableDimensions=1  BreakpointsForDimension1=[0;8.5;17;26;34;42;50;58.3;66.66;85;100]  Table=[370;350;330;310;290;270;250;226;210;186;166.66]  InternalRulePriority=Speed  RndMeth=Simplest
  I : Outport
  V : Outport  Port=2
  wires:
  In1/1 -> Power2I1/1, Power2I/1
  Power2I/1 -> I/1
  Power2I1/1 -> V/1
